simulink model "MsgEthernetMdl"  (R2024a)
settings: Solver=VariableStepAuto  StartTime=0.0  StopTime=50  FixedStep=1  MaxStep=Inf  RelTol=1e-3  EnableMultiTasking=on
PreLoadFcn:
  | load ethernetTypes.mat;
InitFcn:
  | BitRate = 10e6;
undefined symbols (not defined in the file): gateControl, m
settings Model: Creator=The MathWorks, Inc.  LastModifiedBy=uditpant
settings SolverCC: AlgebraicLoopSolver=TrustRegion
settings DataIOCC: ReturnWorkspaceOutputs=off
settings OptimizationCC: LifeSpan=inf
settings DebuggingCC: UnconnectedInputMsg=warning  UnconnectedOutputMsg=warning  UnconnectedLineMsg=warning  SFUnexpectedBacktrackingDiag=warning  SFNoUnconditionalDefaultTransitionDiag=warning  ArithmeticOperatorsInVariantConditions=warning
settings ModelReferenceCC: EnableRefExpFcnMdlSchedulingChecks=on
settings SFSimCC: SimUseLocalCustomCode=off  CustomCodeUndefinedFunction=UseInterfaceOnly
settings RTWCC: RTWUseLocalCustomCode=off  GPUComputeCapability=3.5
settings CodeAppCC: StateflowObjectComments=on
settings GRTTargetCC: TargetLangStandard=C89/C90 (ANSI)
settings ConfigComp: CovMetricSettings=dw  CovSaveCumulativeToWorkspaceVar=on  CovSaveSingleToWorkspaceVar=on  CovExternalEMLEnable=off

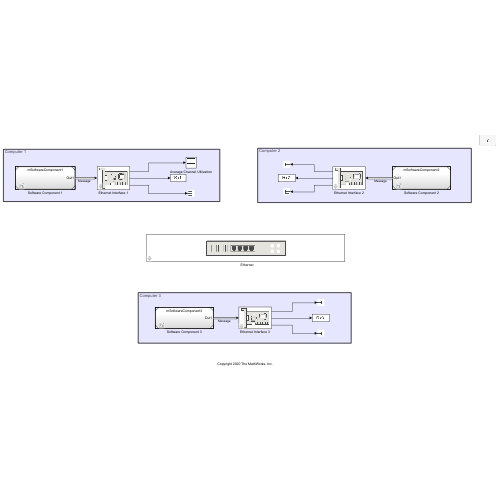
[thumbnail: Simulink's stored preview of the top-level diagram]
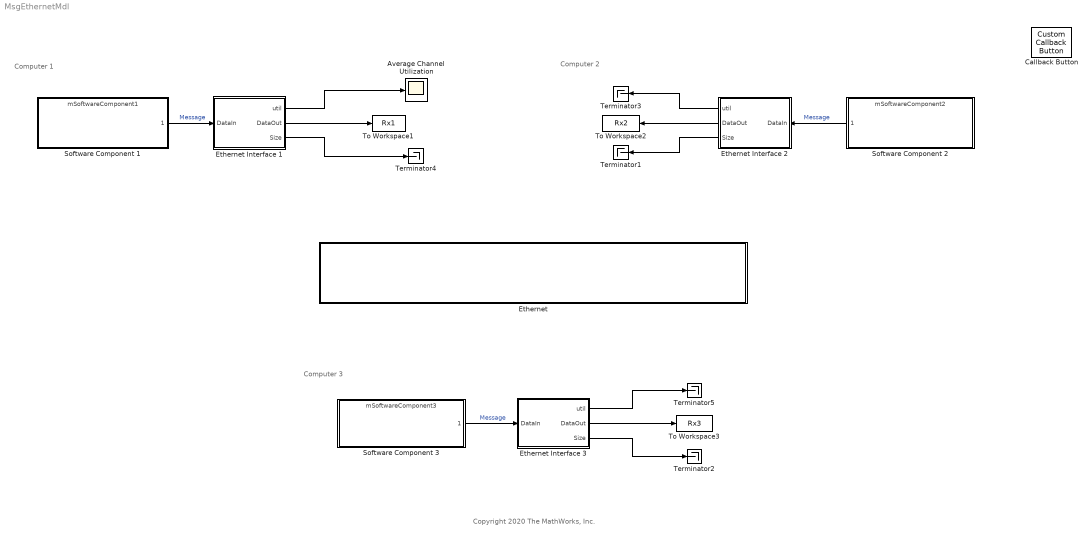
== system MsgEthernetMdl ==
  note: Computer 2
  note: Computer 3
  note: Computer 1
  note: Copyright 2020 The MathWorks, Inc.
  "   Ethernet" : Subsystem  mask(Ethernet Hub){Stations=[3 2 1], CableLength=[200 300 100], PER=[0 0 0], ProcessingTime=0}
      mask prompts: Stations "Connected stations"; CableLength "Length of cables (m)"; PER "Packet error rate (PER)"; ProcessingTime "Processing time (s)"
      mask help: Connect Ethernet stations
      mask init:
      | if length(Stations) < 2
      |     error('Number of connected stations must be greater than 1');
      | end
      | if length(CableLength) ~= length(Stations)
      |     error('Parameter ''Length of cables'' must be a vector with number of elements equals to number of connected stations');
      | end
      | if length(PER) ~= length(Stations)
      |     error('Parameter ''Packet error rate'' must be a vector with number of elements equals to number of connected stations');
      | end
      | ethernetHubMask(gcb, Stations);
      mask DialogControl Container2 Prompt: Parameters
      mask Display: image('ethernet-illustration.png')
  Average Channel Utilization : Scope
  Callback Button : CustomCallbackButton  Configuration="{\"components\":[{\"name\":\"BackgroundImageComponent\",\"settings\":{\"image\":{\"size\":[0,0],\"src\":\"default\",\"srcOrientation\":\"Right\"},\"position\":[0,0,1,1]}},{\"name\":\"ButtonStateComponent\",\"settings\":{\"buttonType\":\"momentary\",\"clickFcn\":\"showExample('simulink\\/EthernetUsingMessagesSimEventsAndStateflowExample')\",\"onValue\":1,\"position\":[0,0,1,1],\"pressDelay\":\"500\",\"pressFcn\":\"\",\"repeatInterval\":\"0\",\"states\":[{\"horizontalAlignment\":\"center\",\"image\":{\"position\":[0,0,1,1],\"src\":\"default\",\"srcOrientation\":\"Right\"},\"label\":{\"color\":[0.01176470588,0.01176470588,0.01176470588,1],\"icon\":{\"size\":[0,0],\"src\":\"default\",\"srcOrientation\":\"Right\"},\"iconPlacement\":\"left\",\"text\":{\"content\":\"?\"}},\"labelOffset\":[0,0],\"verticalAlignment\":\"middle\"},{\"horizontalAlignment\":\"center\",\"image\":{\"position\":[0,0,1,1],\"src\":\"default\",\"srcOrientation\":\"Right\"},\"label\":{\"color\":[0.01176470588,0.01176470588,0.01176470588,1],\"icon\":{\"size\":[0,0],\"src\":\"default\",\"srcOrientation\":\"Right\"},\"iconPlacement\":\"left\",\"text\":{\"content\":\"?\"}},\"labelOffset\":[0,0],\"verticalAlignment\":\"middle\"},{\"horizontalAlignment\":\"center\",\"image\":{\"position\":[0,0,1,1],\"src\":\"default\",\"srcOrientation\":\"Right\"},\"label\":{\"color\":[0.01176470588,0.01176470588,0.01176470588,1],\"icon\":{\"size\":[0,0],\"src\":\"default\",\"srcOrientation\":\"Right\"},\"iconPlacement\":\"left\",\"text\":{\"content\":\"?\"}},\"labelOffset\":[0,0],\"verticalAlignment\":\"middle\"},{\"horizontalAlignment\":\"center\",\"image\":{\"position\":[0,0,1,1],\"src\":\"default\",\"srcOrientation\":\"Right\"},\"label\":{\"color\":[0.01176470588,0.01176470588,0.01176470588,1],\"icon\":{\"size\":[0,0],\"src\":\"default\",\"srcOrientation\":\"Right\"},\"iconPlacement\":\"left\",\"text\":{\"content\":\"?\"}},\"labelOffset\":[0,0],\"verticalAlignment\":\"middle\"}]}},{\"name\":\"ForegroundImageComponent\",\"settings\":{\"image\":{\"size\":[0,0],\"src\":\"default\",\"srcOrientation\":\"Right\"},\"isForeground\":1,\"position\":[0,0,1,1]}}],\"settings\":{\"BindingType\":\"standalone\",\"backgroundColor\":[244,244,244,1],\"backgroundOffset\":0.2,\"backgroundOpacity\":1,\"fixedAspectRatio\":\"off\",\"foregroundColor\":[0.01176470588,0.01176470588,0.01176470588,1],\"migratedFromLegacy\":true,\"useBackgroundColor\":true,\"variant\":\"callback\",\"version\":\"R2023a\"},\"type\":\"Button\"}"  CustomBackgroundColor="{\"color\":[0.9568627451,0.9568627451,0.9568627451],\"show\":true}"
  Ethernet Interface 1 : Subsystem  mask(Ethernet MAC Layer){StationID=1, TxBufferCapacity=256}
      mask prompts: StationID "Station ID"; TxBufferCapacity "Transmission buffer capacity"
      mask help: Ethernet MAC layer packet transmission and reception based on CSMA/CD
      mask init:
      | ethernetStationMask(gcb, StationID);
      mask Display: image('ethernet-interface-illustration.png')
  Ethernet Interface 2 : Subsystem  mask(Ethernet MAC Layer){StationID=2, TxBufferCapacity=256}
      mask prompts: StationID "Station ID"; TxBufferCapacity "Transmission buffer capacity"
      mask help: Ethernet MAC layer packet transmission and reception based on CSMA/CD
      mask init:
      | ethernetStationMask(gcb, StationID);
      mask Display: image('ethernet-interface-illustration.png')
  Ethernet Interface 3 : Subsystem  mask(Ethernet MAC Layer){StationID=3, TxBufferCapacity=256}
      mask prompts: StationID "Station ID"; TxBufferCapacity "Transmission buffer capacity"
      mask help: Ethernet MAC layer packet transmission and reception based on CSMA/CD
      mask init:
      | ethernetStationMask(gcb, StationID);
      mask Display: image('ethernet-interface-illustration.png')
  Software Component 1 : ModelReference  OutputPortMessageModes=m  ModelNameDialog=mSoftwareComponent1  SimulationMode=Normal  ModelReferenceVersion=9.0
  Software Component 2 : ModelReference  OutputPortMessageModes=m  ModelNameDialog=mSoftwareComponent2  SimulationMode=Normal  ModelReferenceVersion=9.0
  Software Component 3 : ModelReference  OutputPortMessageModes=m  ModelNameDialog=mSoftwareComponent3  SimulationMode=Normal  ModelReferenceVersion=9.0
  Terminator{1..5} (5 alike) : Terminator
  To Workspace1 : ToWorkspace  VariableName=Rx1  SaveFormat=Timeseries  SampleTime=-1
  To Workspace2 : ToWorkspace  VariableName=Rx2  SaveFormat=Timeseries  SampleTime=-1
  To Workspace3 : ToWorkspace  VariableName=Rx3  SaveFormat=Timeseries  SampleTime=-1
  wires:
  Ethernet Interface 1/2(DataOut) -> To Workspace1/1
  Ethernet Interface 1/1(util) -> Average Channel Utilization/1
  Ethernet Interface 1/3(Size) -> Terminator4/1
  Software Component 1/1 -> Ethernet Interface 1/1(DataIn)  "Message"
  Software Component 2/1 -> Ethernet Interface 2/1(DataIn)  "Message"
  Software Component 3/1 -> Ethernet Interface 3/1(DataIn)  "Message"
  Ethernet Interface 2/2(DataOut) -> To Workspace2/1
  Ethernet Interface 2/3(Size) -> Terminator1/1
  Ethernet Interface 2/1(util) -> Terminator3/1
  Ethernet Interface 3/2(DataOut) -> To Workspace3/1
  Ethernet Interface 3/3(Size) -> Terminator2/1
  Ethernet Interface 3/1(util) -> Terminator5/1

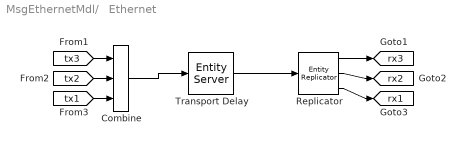
== system MsgEthernetMdl/   Ethernet ==
  Combine : EntityInputSwitch  InputPortMessageModes=m,m,m  OutputPortMessageModes=m  NumberInputPorts=3
      settings: InputPortMap=u1,u2,u3
  Replicator : EntityReplicator  InputPortMessageModes=m  OutputPortMessageModes=m,m,m  NumberReplicas=2
      settings: OutputPortMap=o0,o1,o2
  Transport Delay : EntityServer  InputPortMessageModes=m  OutputPortMessageModes=m  Capacity=Inf  ServiceTimeSource=MATLAB action  ServiceTimeAction=|  ServiceCompleteAction=|
      ServiceTimeAction=|
      | src = entity.TxAddress;
      | dst = entity.RxAddress;
      | srcl = 0;
      | dstl = 0;
      | for i = 1:length(Stations)
      |     if src == Stations(i)
      |         srcl = CableLength(i);
      |     end
      |     if dst == Stations(i)
      |         dstl = CableLength(i);
      |     end
      |     if srcl > 0 && dstl > 0
      |         break;
      |     end
      | end
      | dt = ProcessingTime + (srcl + dstl)/3e8;
      ServiceCompleteAction=|
      | src = entity.TxAddress;
      | dst = entity.RxAddress;
      | srcIdx = 0;
      | dstIdx = 0;
      | for i = 1:length(Stations)
      |     if src == Stations(i)
      |         srcIdx = i;
      |     end
      |     if dst == Stations(i)
      |         dstIdx = i;
      |     end
      |     if srcIdx > 0 && dstIdx > 0
      |         break;
      |     end
      | end
      | if rand < (PER(srcIdx) + PER(dstIdx))
      |     entity.CRC = 1;
      | end
  tag scope: rx1=global, rx2=global, rx3=global
  wires:
  Combine/1 -> Transport Delay/1
  Transport Delay/1 -> Replicator/1
  [tx3] -> Combine/1
  Replicator/1 -> [rx3]
  [tx2] -> Combine/2
  Replicator/2 -> [rx2]
  [tx1] -> Combine/3
  Replicator/3 -> [rx1]

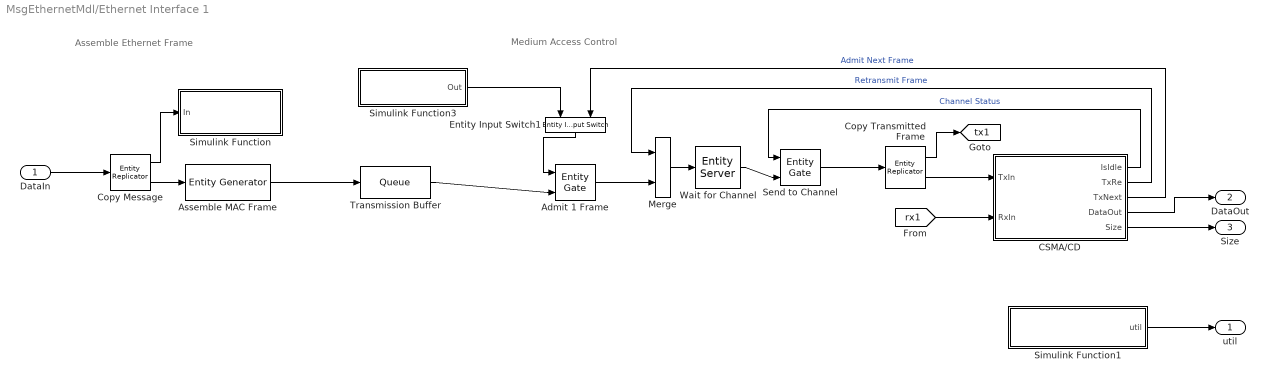
== system MsgEthernetMdl/Ethernet Interface 1 ==
  note: Assemble Ethernet Frame
  note: Medium Access Control
  DataIn : Inport
  "Admit 1 Frame " : EntityGate  InputPortMessageModes=m,m  OutputPortMessageModes=m  OpenGateAtSimulationStart=on
  Assemble MAC Frame : EntityGenerator  InputPortMessageModes=m  OutputPortMessageModes=m  GenerationMethod=Event-based  GenerateAction=|  EntityType=Bus object  EntityTypeName=ethernetPacket
      | entity.TxAddress = StationID;
      | [entity.RxAddress, entity.Data, entity.PayloadSize] = ...
      |     initPacket();
      | entity.TxDelay = (entity.PayloadSize+22)*8/BitRate;
      | entity.BackoffTime = 0;
      | entity.CRC = 0;
      settings: InputPortMap=u0
  CSMA/CD : Stateflow chart  TreatAsAtomicUnit=on
  Copy Message : EntityReplicator  InputPortMessageModes=m  OutputPortMessageModes=m,m
  Copy Transmitted Frame : EntityReplicator  InputPortMessageModes=m  OutputPortMessageModes=m,m
  Entity Input Switch1 : EntityInputSwitch  InputPortMessageModes=m,m  OutputPortMessageModes=m
  "Merge " : EntityInputSwitch  InputPortMessageModes=m,m  OutputPortMessageModes=m
  Send to Channel : EntityGate  InputPortMessageModes=m,m  OutputPortMessageModes=m  OpenGateAtSimulationStart=on
  Simulink Function : Subsystem  TreatAsAtomicUnit=on
  Simulink Function1 : Subsystem  TreatAsAtomicUnit=on
  Simulink Function3 : Subsystem  TreatAsAtomicUnit=on
  Transmission Buffer : Queue  InputPortMessageModes=m  OutputPortMessageModes=m  Capacity=TxBufferCapacity  ExitAction=gateControl();
  Wait for Channel : EntityServer  InputPortMessageModes=m  OutputPortMessageModes=m  Capacity=1  ServiceTimeSource=Attribute  ServiceTimeAttributeName=BackoffTime
  util : Outport
  DataOut : Outport  Port=2
  Size : Outport  Port=3
  tag scope: tx1=global
  wires:
  CSMA/CD/5(Size) -> Size/1
  Simulink Function1/1(util) -> util/1
  CSMA/CD/4(DataOut) -> DataOut/1
  CSMA/CD/1(IsIdle) -> Send to Channel/1  "Channel Status"
  CSMA/CD/3(TxNext) -> Entity Input Switch1/2  "Admit Next Frame"
  Transmission Buffer/1 -> "Admit 1 Frame "/2
  "Admit 1 Frame "/1 -> "Merge "/2
  "Merge "/1 -> Wait for Channel/1
  Wait for Channel/1 -> Send to Channel/2
  Send to Channel/1 -> Copy Transmitted Frame/1
  Copy Transmitted Frame/2 -> CSMA/CD/1(TxIn)
  [rx1] -> CSMA/CD/2(RxIn)
  CSMA/CD/2(TxRe) -> "Merge "/1  "Retransmit Frame"
  Copy Transmitted Frame/1 -> [tx1]
  Assemble MAC Frame/1 -> Transmission Buffer/1
  DataIn/1 -> Copy Message/1
  Copy Message/2 -> Assemble MAC Frame/1
  Copy Message/1 -> Simulink Function/1(In)
  Entity Input Switch1/1 -> "Admit 1 Frame "/1
  Simulink Function3/1(Out) -> Entity Input Switch1/1

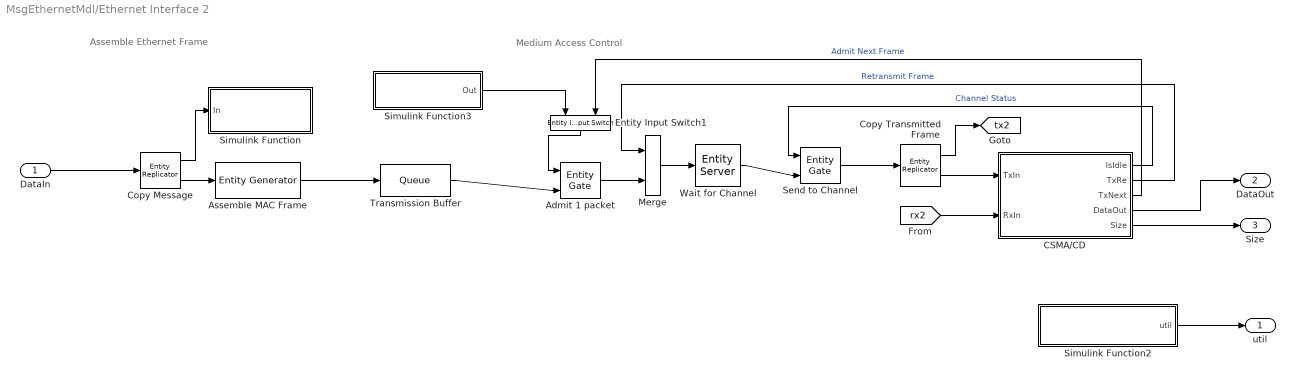
== system MsgEthernetMdl/Ethernet Interface 2 ==
  note: Medium Access Control
  note: Assemble Ethernet Frame
  DataIn : Inport
  "Admit 1 packet " : EntityGate  InputPortMessageModes=m,m  OutputPortMessageModes=m  OpenGateAtSimulationStart=on
  Assemble MAC Frame : EntityGenerator  InputPortMessageModes=m  OutputPortMessageModes=m  GenerationMethod=Event-based  GenerateAction=|  EntityType=Bus object  EntityTypeName=ethernetPacket
      | entity.TxAddress = StationID;
      | [entity.RxAddress, entity.Data, entity.PayloadSize] = ...
      |     initPacket();
      | entity.TxDelay = (entity.PayloadSize+22)*8/BitRate;
      | entity.BackoffTime = 0;
      | entity.CRC = 0;
      settings: InputPortMap=u0
  CSMA/CD : Stateflow chart  TreatAsAtomicUnit=on
  Copy Message : EntityReplicator  InputPortMessageModes=m  OutputPortMessageModes=m,m
  Copy Transmitted Frame : EntityReplicator  InputPortMessageModes=m  OutputPortMessageModes=m,m
  Entity Input Switch1 : EntityInputSwitch  InputPortMessageModes=m,m  OutputPortMessageModes=m
  Merge : EntityInputSwitch  InputPortMessageModes=m,m  OutputPortMessageModes=m
  Send to Channel : EntityGate  InputPortMessageModes=m,m  OutputPortMessageModes=m  OpenGateAtSimulationStart=on
  Simulink Function : Subsystem  TreatAsAtomicUnit=on
  Simulink Function2 : Subsystem  TreatAsAtomicUnit=on
  Simulink Function3 : Subsystem  TreatAsAtomicUnit=on
  Transmission Buffer : Queue  InputPortMessageModes=m  OutputPortMessageModes=m  Capacity=TxBufferCapacity  ExitAction=gateControl();
  Wait for Channel : EntityServer  InputPortMessageModes=m  OutputPortMessageModes=m  Capacity=1  ServiceTimeSource=Attribute  ServiceTimeAttributeName=BackoffTime
  util : Outport
  DataOut : Outport  Port=2
  Size : Outport  Port=3
  tag scope: tx2=global
  wires:
  CSMA/CD/5(Size) -> Size/1
  Simulink Function2/1(util) -> util/1
  CSMA/CD/4(DataOut) -> DataOut/1
  CSMA/CD/1(IsIdle) -> Send to Channel/1  "Channel Status"
  CSMA/CD/3(TxNext) -> Entity Input Switch1/2  "Admit Next Frame"
  Transmission Buffer/1 -> "Admit 1 packet "/2
  "Admit 1 packet "/1 -> Merge/2
  Merge/1 -> Wait for Channel/1
  Wait for Channel/1 -> Send to Channel/2
  Send to Channel/1 -> Copy Transmitted Frame/1
  Copy Transmitted Frame/2 -> CSMA/CD/1(TxIn)
  [rx2] -> CSMA/CD/2(RxIn)
  CSMA/CD/2(TxRe) -> Merge/1  "Retransmit Frame"
  Copy Transmitted Frame/1 -> [tx2]
  Assemble MAC Frame/1 -> Transmission Buffer/1
  DataIn/1 -> Copy Message/1
  Copy Message/2 -> Assemble MAC Frame/1
  Copy Message/1 -> Simulink Function/1(In)
  Simulink Function3/1(Out) -> Entity Input Switch1/1
  Entity Input Switch1/1 -> "Admit 1 packet "/1

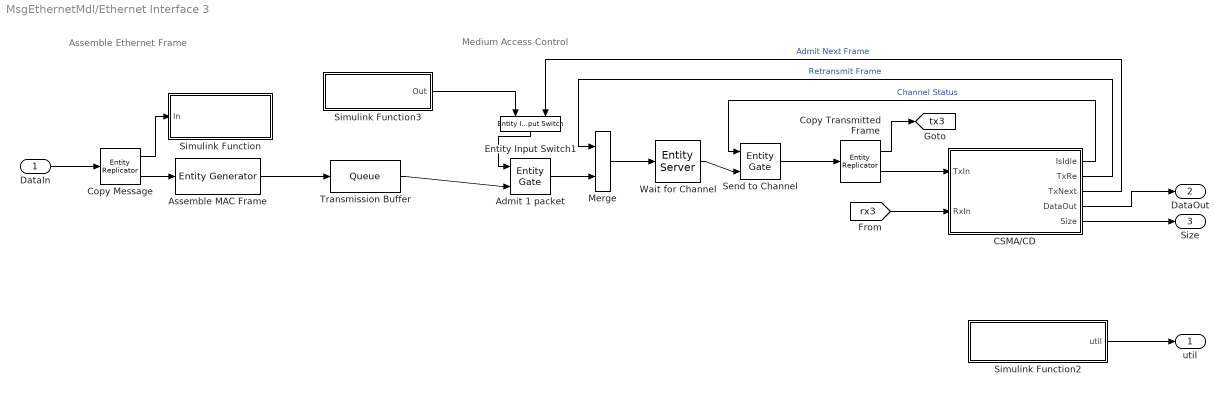
== system MsgEthernetMdl/Ethernet Interface 3 ==
  note: Medium Access Control
  note: Assemble Ethernet Frame
  DataIn : Inport
  "Admit 1 packet " : EntityGate  InputPortMessageModes=m,m  OutputPortMessageModes=m  OpenGateAtSimulationStart=on
  Assemble MAC Frame : EntityGenerator  InputPortMessageModes=m  OutputPortMessageModes=m  GenerationMethod=Event-based  GenerateAction=|  EntityType=Bus object  EntityTypeName=ethernetPacket
      | entity.TxAddress = StationID;
      | [entity.RxAddress, entity.Data, entity.PayloadSize] = ...
      |     initPacket();
      | entity.TxDelay = (entity.PayloadSize+22)*8/BitRate;
      | entity.BackoffTime = 0;
      | entity.CRC = 0;
      settings: InputPortMap=u0
  CSMA/CD : Stateflow chart  TreatAsAtomicUnit=on
  Copy Message : EntityReplicator  InputPortMessageModes=m  OutputPortMessageModes=m,m
  Copy Transmitted Frame : EntityReplicator  InputPortMessageModes=m  OutputPortMessageModes=m,m
  Entity Input Switch1 : EntityInputSwitch  InputPortMessageModes=m,m  OutputPortMessageModes=m
  Merge : EntityInputSwitch  InputPortMessageModes=m,m  OutputPortMessageModes=m
  Send to Channel : EntityGate  InputPortMessageModes=m,m  OutputPortMessageModes=m  OpenGateAtSimulationStart=on
  Simulink Function : Subsystem  TreatAsAtomicUnit=on
  Simulink Function2 : Subsystem  TreatAsAtomicUnit=on
  Simulink Function3 : Subsystem  TreatAsAtomicUnit=on
  Transmission Buffer : Queue  InputPortMessageModes=m  OutputPortMessageModes=m  Capacity=TxBufferCapacity  ExitAction=gateControl();
  Wait for Channel : EntityServer  InputPortMessageModes=m  OutputPortMessageModes=m  Capacity=1  ServiceTimeSource=Attribute  ServiceTimeAttributeName=BackoffTime
  util : Outport
  DataOut : Outport  Port=2
  Size : Outport  Port=3
  tag scope: tx3=global
  wires:
  CSMA/CD/5(Size) -> Size/1
  Simulink Function2/1(util) -> util/1
  CSMA/CD/4(DataOut) -> DataOut/1
  CSMA/CD/1(IsIdle) -> Send to Channel/1  "Channel Status"
  CSMA/CD/3(TxNext) -> Entity Input Switch1/2  "Admit Next Frame"
  Transmission Buffer/1 -> "Admit 1 packet "/2
  "Admit 1 packet "/1 -> Merge/2
  Merge/1 -> Wait for Channel/1
  Wait for Channel/1 -> Send to Channel/2
  Send to Channel/1 -> Copy Transmitted Frame/1
  Copy Transmitted Frame/2 -> CSMA/CD/1(TxIn)
  [rx3] -> CSMA/CD/2(RxIn)
  CSMA/CD/2(TxRe) -> Merge/1  "Retransmit Frame"
  Copy Transmitted Frame/1 -> [tx3]
  Assemble MAC Frame/1 -> Transmission Buffer/1
  DataIn/1 -> Copy Message/1
  Copy Message/2 -> Assemble MAC Frame/1
  Copy Message/1 -> Simulink Function/1(In)
  Entity Input Switch1/1 -> "Admit 1 packet "/1
  Simulink Function3/1(Out) -> Entity Input Switch1/1

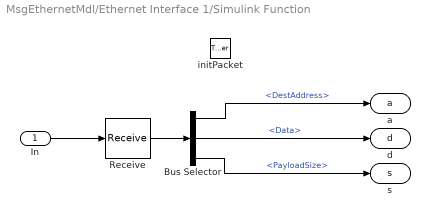
== system MsgEthernetMdl/Ethernet Interface 1/Simulink Function ==
  In : Inport
  initPacket : TriggerPort  TriggerType=function-call  IsSimulinkFunction=on  FunctionName=initPacket  FunctionVisibility=scoped  VariantControl=(inherit)
  Bus Selector : BusSelector  OutputSignals=DestAddress,Data,PayloadSize
  Receive : Receive  InputPortMessageModes=m  QueueLength=2^16-1
  a : ArgOut  DisableCoverage=on  ArgumentName=a
  d : ArgOut  Port=2  PortDimensions=[1 1500]  ArgumentName=d
  s : ArgOut  Port=3  ArgumentName=s
  wires:
  Bus Selector/3 -> s/1  "<PayloadSize>"
  Bus Selector/2 -> d/1  "<Data>"
  Receive/1 -> Bus Selector/1
  In/1 -> Receive/1
  Bus Selector/1 -> a/1  "<DestAddress>"

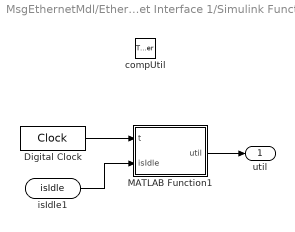
== system MsgEthernetMdl/Ethernet Interface 1/Simulink Function1 ==
  compUtil : TriggerPort  TriggerType=function-call  IsSimulinkFunction=on  FunctionName=compUtil  FunctionVisibility=scoped  VariantControl=(inherit)
  Digital Clock : DigitalClock  SampleTime=-1
  MATLAB Function1 : MATLAB Function  TreatAsAtomicUnit=on
  isIdle1 : ArgIn  ArgumentName=isIdle
  util : Outport
  wires:
  Digital Clock/1 -> MATLAB Function1/1(t)
  isIdle1/1 -> MATLAB Function1/2(isIdle)
  MATLAB Function1/1(util) -> util/1

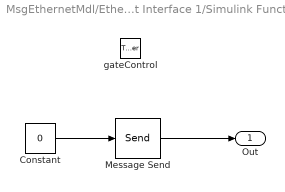
== system MsgEthernetMdl/Ethernet Interface 1/Simulink Function3 ==
  gateControl : TriggerPort  TriggerType=function-call  IsSimulinkFunction=on  FunctionName=gateControl  FunctionVisibility=scoped  VariantControl=Variant
  Constant : Constant  Value=0
  Message Send : Send  OutputPortMessageModes=m
  Out : Outport
  wires:
  Message Send/1 -> Out/1
  Constant/1 -> Message Send/1

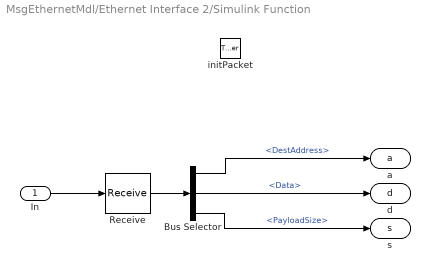
== system MsgEthernetMdl/Ethernet Interface 2/Simulink Function ==
  In : Inport
  initPacket : TriggerPort  TriggerType=function-call  IsSimulinkFunction=on  FunctionName=initPacket  FunctionVisibility=scoped  VariantControl=(inherit)
  Bus Selector : BusSelector  OutputSignals=DestAddress,Data,PayloadSize
  Receive : Receive  InputPortMessageModes=m  QueueLength=2^16-1
  a : ArgOut  DisableCoverage=on  ArgumentName=a
  d : ArgOut  Port=2  PortDimensions=[1 1500]  ArgumentName=d
  s : ArgOut  Port=3  ArgumentName=s
  wires:
  Bus Selector/3 -> s/1  "<PayloadSize>"
  Bus Selector/2 -> d/1  "<Data>"
  Receive/1 -> Bus Selector/1
  In/1 -> Receive/1
  Bus Selector/1 -> a/1  "<DestAddress>"

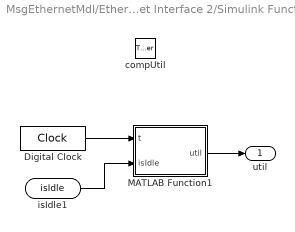
== system MsgEthernetMdl/Ethernet Interface 2/Simulink Function2 ==
  compUtil : TriggerPort  TriggerType=function-call  IsSimulinkFunction=on  FunctionName=compUtil  FunctionVisibility=scoped  VariantControl=(inherit)
  Digital Clock : DigitalClock  SampleTime=-1
  MATLAB Function1 : MATLAB Function  TreatAsAtomicUnit=on
  isIdle1 : ArgIn  ArgumentName=isIdle
  util : Outport
  wires:
  Digital Clock/1 -> MATLAB Function1/1(t)
  isIdle1/1 -> MATLAB Function1/2(isIdle)
  MATLAB Function1/1(util) -> util/1

== system MsgEthernetMdl/Ethernet Interface 2/Simulink Function3 ==
  gateControl : TriggerPort  TriggerType=function-call  IsSimulinkFunction=on  FunctionName=gateControl  FunctionVisibility=scoped  VariantControl=Variant
  Constant : Constant  Value=0
  Message Send : Send  OutputPortMessageModes=m
  Out : Outport
  wires:
  Message Send/1 -> Out/1
  Constant/1 -> Message Send/1

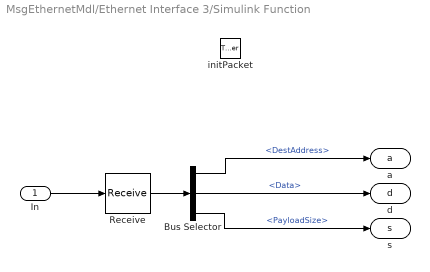
== system MsgEthernetMdl/Ethernet Interface 3/Simulink Function ==
  In : Inport
  initPacket : TriggerPort  TriggerType=function-call  IsSimulinkFunction=on  FunctionName=initPacket  FunctionVisibility=scoped  VariantControl=(inherit)
  Bus Selector : BusSelector  OutputSignals=DestAddress,Data,PayloadSize
  Receive : Receive  InputPortMessageModes=m  QueueLength=2^16-1
  a : ArgOut  DisableCoverage=on  ArgumentName=a
  d : ArgOut  Port=2  PortDimensions=[1 1500]  ArgumentName=d
  s : ArgOut  Port=3  ArgumentName=s
  wires:
  Bus Selector/3 -> s/1  "<PayloadSize>"
  Bus Selector/2 -> d/1  "<Data>"
  Receive/1 -> Bus Selector/1
  In/1 -> Receive/1
  Bus Selector/1 -> a/1  "<DestAddress>"

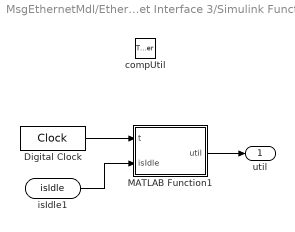
== system MsgEthernetMdl/Ethernet Interface 3/Simulink Function2 ==
  compUtil : TriggerPort  TriggerType=function-call  IsSimulinkFunction=on  FunctionName=compUtil  FunctionVisibility=scoped  VariantControl=(inherit)
  Digital Clock : DigitalClock  SampleTime=-1
  MATLAB Function1 : MATLAB Function  TreatAsAtomicUnit=on
  isIdle1 : ArgIn  ArgumentName=isIdle
  util : Outport
  wires:
  Digital Clock/1 -> MATLAB Function1/1(t)
  isIdle1/1 -> MATLAB Function1/2(isIdle)
  MATLAB Function1/1(util) -> util/1

== system MsgEthernetMdl/Ethernet Interface 3/Simulink Function3 ==
  gateControl : TriggerPort  TriggerType=function-call  IsSimulinkFunction=on  FunctionName=gateControl  FunctionVisibility=scoped  VariantControl=Variant
  Constant : Constant  Value=0
  Message Send : Send  OutputPortMessageModes=m
  Out : Outport
  wires:
  Message Send/1 -> Out/1
  Constant/1 -> Message Send/1

== stateflow chart MsgEthernetMdl/Ethernet Interface 2/CSMA//CD ==
  settings: enableNonTerminalStates=1
  state Standby
    en:
    IsIdle.data = 1;
    send(IsIdle);
    compUtil(1);
  state Receiving
    en:
    delay = RxIn.data.TxDelay;
    err = RxIn.data.CRC;
    forward(RxIn, Rx);
    IsIdle.data = 0;
    send(IsIdle);
    compUtil(0);
  state Transmitting
    en:
    delay = TxIn.data.TxDelay;
    forward(TxIn, TxBuffer);
    IsIdle.data = 0;
    send(IsIdle);
    compUtil(0);
  state Collision
    en:
    n = n + 1;
  state TxSuccess
  state RxSuccess
  state RxFail
  state TxReset
  state RxReset
  (default) -> Standby : {InitRand(); n = 0;}
  TxReset -> Standby
  RxReset -> Standby
  Standby -> Receiving [order 2] : RxIn
  Standby -> Transmitting [order 1] : TxIn
  Transmitting -> TxSuccess [order 1] : after(delay, sec)
  Transmitting -> Collision [order 2] : RxIn[RxIn.data.TxAddress ~= StationID]
  Receiving -> RxFail [order 1] : RxIn
  Receiving -> (junction 14) [order 2] : after(delay, sec)
  (junction 14) -> RxFail [order 2]
  (junction 14) -> RxSuccess [order 1] : [err == 0]
  TxSuccess -> TxReset : TxBuffer
      | {n = 0; TxNext.data=1;
      | send(TxNext);}
  RxSuccess -> (junction 1) : Rx
  RxFail -> RxReset : Rx
  Collision -> (junction 7) : TxBuffer
  (junction 1) -> RxReset [order 1] : [Rx.data.RxAddress == StationID]
      | {DataOut.data = Rx.data.Data;
      | Size = Rx.data.PayloadSize;
      | send(DataOut);}
  (junction 1) -> RxReset [order 2]
  (junction 7) -> TxReset [order 2] : {n = 0;TxNext.data=1;
      |  send(TxNext);}
  (junction 7) -> TxReset [order 1] : [n<16] {TxBuffer.data.BackoffTime = Backoff(n);
      |              forward(TxBuffer, TxRe);}
  data: u function_input; t function_output; IsIdle output double size=1; TxRe output Bus: ethernetPacket size=1; TxNext output double size=1; TxIn input Bus: ethernetPacket size=1; DataOut output double size=[1 1500]; RxIn input Bus: ethernetPacket size=1; delay local double size=1; n local double size=1; TxBuffer local Bus: ethernetPacket size=1; Rx local Bus: ethernetPacket size=1; err local double; StationID parameter; Size output double size=1
  function t = Backoff(u):
    | function t = Backoff(u)
    | t = floor(rand*(2^min([u,10])))*5.12e-5;
  function InitRand:
    | function InitRand
    | rand('seed', StationID);

== matlab function MsgEthernetMdl/Ethernet Interface 2/Simulink Function2/MATLAB Function1 ==
  data: t input; util output; isIdle input
function util = fcn(t, isIdle)

persistent lastTime lastState totalUse;

if isempty(lastTime)
    lastTime = 0;
    lastState = 0;
    totalUse = 0;
end

if lastState ==1 % busy
    totalUse = totalUse + (t - lastTime);
end
lastTime = t;
if isIdle
    lastState = 0;
else
    lastState = 1;
end
if t > 0
    util = totalUse/t;
else
    util = lastState;
end

== stateflow chart MsgEthernetMdl/Ethernet Interface 1/CSMA//CD ==
  settings: enableNonTerminalStates=1
  state Standby
    en:
    IsIdle.data = 1;
    send(IsIdle);
    compUtil(1);
  state Receiving
    en:
    delay = RxIn.data.TxDelay;
    err = RxIn.data.CRC;
    forward(RxIn, Rx);
    IsIdle.data = 0;
    send(IsIdle);
    compUtil(0);
  state Transmitting
    en:
    delay = TxIn.data.TxDelay;
    forward(TxIn, TxBuffer);
    IsIdle.data = 0;
    send(IsIdle);
    compUtil(0);
  state Collision
    en:
    n = n + 1;
  state TxSuccess
  state RxSuccess
  state RxFail
  state TxReset
  state RxReset
  (default) -> Standby : {InitRand(); n = 0;}
  TxReset -> Standby
  RxReset -> Standby
  Standby -> Receiving [order 2] : RxIn
  Standby -> Transmitting [order 1] : TxIn
  Transmitting -> TxSuccess [order 1] : after(delay, sec)
  Transmitting -> Collision [order 2] : RxIn[RxIn.data.TxAddress ~= StationID]
  Receiving -> RxFail [order 1] : RxIn
  Receiving -> (junction 14) [order 2] : after(delay, sec)
  (junction 14) -> RxFail [order 2]
  (junction 14) -> RxSuccess [order 1] : [err == 0]
  TxSuccess -> TxReset : TxBuffer
      | {n = 0; TxNext.data=1;
      | send(TxNext);}
  RxSuccess -> (junction 1) : Rx
  RxFail -> RxReset : Rx
  Collision -> (junction 7) : TxBuffer
  (junction 1) -> RxReset [order 1] : [Rx.data.RxAddress == StationID]
      | {DataOut.data = Rx.data.Data;
      | Size = Rx.data.PayloadSize;
      | send(DataOut);}
  (junction 1) -> RxReset [order 2]
  (junction 7) -> TxReset [order 2] : {n = 0;TxNext.data=1;
      |  send(TxNext);}
  (junction 7) -> TxReset [order 1] : [n<16] {TxBuffer.data.BackoffTime = Backoff(n);
      |              forward(TxBuffer, TxRe);}
  data: u function_input; t function_output; IsIdle output double size=1; TxRe output Bus: ethernetPacket size=1; TxNext output double size=1; TxIn input Bus: ethernetPacket size=1; DataOut output double size=[1 1500]; RxIn input Bus: ethernetPacket size=1; delay local double size=1; n local double size=1; TxBuffer local Bus: ethernetPacket size=1; Rx local Bus: ethernetPacket size=1; err local double; StationID parameter; Size output double size=1
  function t = Backoff(u):
    | function t = Backoff(u)
    | t = floor(rand*(2^min([u,10])))*5.12e-5;
  function InitRand:
    | function InitRand
    | rand('seed', StationID);

== matlab function MsgEthernetMdl/Ethernet Interface 3/Simulink Function2/MATLAB Function1 ==
  data: t input; util output; isIdle input
function util = fcn(t, isIdle)

persistent lastTime lastState totalUse;

if isempty(lastTime)
    lastTime = 0;
    lastState = 0;
    totalUse = 0;
end

if lastState ==1 % busy
    totalUse = totalUse + (t - lastTime);
end
lastTime = t;
if isIdle
    lastState = 0;
else
    lastState = 1;
end
if t > 0
    util = totalUse/t;
else
    util = lastState;
end

== matlab function MsgEthernetMdl/Ethernet Interface 1/Simulink Function1/MATLAB Function1 ==
  data: t input; util output; isIdle input
function util = fcn(t, isIdle)

persistent lastTime lastState totalUse;

if isempty(lastTime)
    lastTime = 0;
    lastState = 0;
    totalUse = 0;
end

if lastState ==1 % busy
    totalUse = totalUse + (t - lastTime);
end
lastTime = t;
if isIdle
    lastState = 0;
else
    lastState = 1;
end
if t > 0
    util = totalUse/t;
else
    util = lastState;
end

== stateflow chart MsgEthernetMdl/Ethernet Interface 3/CSMA//CD ==
  settings: enableNonTerminalStates=1
  state Standby
    en:
    IsIdle.data = 1;
    send(IsIdle);
    compUtil(1);
  state Receiving
    en:
    delay = RxIn.data.TxDelay;
    err = RxIn.data.CRC;
    forward(RxIn, Rx);
    IsIdle.data = 0;
    send(IsIdle);
    compUtil(0);
  state Transmitting
    en:
    delay = TxIn.data.TxDelay;
    forward(TxIn, TxBuffer);
    IsIdle.data = 0;
    send(IsIdle);
    compUtil(0);
  state Collision
    en:
    n = n + 1;
  state TxSuccess
  state RxSuccess
  state RxFail
  state TxReset
  state RxReset
  (default) -> Standby : {InitRand(); n = 0;}
  TxReset -> Standby
  RxReset -> Standby
  Standby -> Receiving [order 2] : RxIn
  Standby -> Transmitting [order 1] : TxIn
  Transmitting -> TxSuccess [order 1] : after(delay, sec)
  Transmitting -> Collision [order 2] : RxIn[RxIn.data.TxAddress ~= StationID]
  Receiving -> RxFail [order 1] : RxIn
  Receiving -> (junction 14) [order 2] : after(delay, sec)
  (junction 14) -> RxFail [order 2]
  (junction 14) -> RxSuccess [order 1] : [err == 0]
  TxSuccess -> TxReset : TxBuffer
      | {n = 0; TxNext.data=1;
      | send(TxNext);}
  RxSuccess -> (junction 1) : Rx
  RxFail -> RxReset : Rx
  Collision -> (junction 7) : TxBuffer
  (junction 1) -> RxReset [order 1] : [Rx.data.RxAddress == StationID]
      | {DataOut.data = Rx.data.Data;
      | Size = Rx.data.PayloadSize;
      | send(DataOut);}
  (junction 1) -> RxReset [order 2]
  (junction 7) -> TxReset [order 2] : {n = 0;TxNext.data=1;
      |  send(TxNext);}
  (junction 7) -> TxReset [order 1] : [n<16] {TxBuffer.data.BackoffTime = Backoff(n);
      |              forward(TxBuffer, TxRe);}
  data: u function_input; t function_output; IsIdle output double size=1; TxRe output Bus: ethernetPacket size=1; TxNext output double size=1; TxIn input Bus: ethernetPacket size=1; DataOut output double size=[1 1500]; RxIn input Bus: ethernetPacket size=1; delay local double size=1; n local double size=1; TxBuffer local Bus: ethernetPacket size=1; Rx local Bus: ethernetPacket size=1; err local double; StationID parameter; Size output double size=1
  function t = Backoff(u):
    | function t = Backoff(u)
    | t = floor(rand*(2^min([u,10])))*5.12e-5;
  function InitRand:
    | function InitRand
    | rand('seed', StationID);
